simulink model "e8_IPMSM_HWJandVent_ROM"  (R2021b)
settings: Solver=VariableStepAuto  StartTime=0.0  StopTime=1000  RelTol=1e-3  AbsTol=1e-3
model workspace (MAT data in the model file):
  AdjacencyMat = [0 0 0 0 0 0 0 0 0 0 0 0 ... (15129 elements, 123x123)]
  Banding_Loss_Mat = [0 0 0 0 0 0 0 0 0 0 0 0 ... (7020 elements, 39x60x3)]
  CapMat = [1e+20 2196.70091586 387.653102799 193.8265514 1962.34710525 387.653102799 193.8265514 1962.34710525 1266.59353814 268.053957132 416.539515956 175.715078 ... (123 elements, 123x1)]
  CoolantArrayIdxs = [20 21 22 23 24 25 26 27 35 36 37 84 ... (19 elements, 19x1)]
  DCBusVoltageVec = [200 300 400]
  Friction_Loss_Mat = [0 0 0 0 0 0 0 0 0 0 0 0 ... (7020 elements, 39x60x3)]
  InletCoolIdxs = [38; 37]
  Iron_Loss_Rotor_Back_Iron_Mat = [0.0117705351991 0.0204390240307 0.0248508325185 0.0256457032681 0.0238785055856 0.020530699908 0.0166089076031 0.0132296142351 0.0115805086727 0.0121981902442 0.0144548234671 0.0172622621719 ... (7020 elements, 39x60x3)]
  Iron_Loss_Rotor_Pole_Mat = [1.45649756865 1.45220158629 1.42754923451 1.38825604934 1.33915333349 1.28386605183 1.22530180492 1.16593914393 1.10785564554 1.05188090135 0.997097257278 0.941639677474 ... (7020 elements, 39x60x3)]
  Iron_Loss_Rotor_Tooth_Mat = [0 0 0 0 0 0 0 0 0 0 0 0 ... (7020 elements, 39x60x3)]
  Iron_Loss_Stator_Back_Iron_Mat = [38.5419456951 37.7152025365 36.7151009719 35.6149517682 34.4520386289 33.2585547415 32.0665067995 30.91142079 29.8301048499 28.8255844376 27.8319778373 26.7434652419 ... (7020 elements, 39x60x3)]
  Iron_Loss_Stator_Tooth_Mat = [42.0610884508 40.9832240847 40.1258499541 39.3817529075 38.6582544091 37.9130136221 37.1370624807 36.3449214788 35.5617649366 34.7840580455 33.951564889 32.9872940506 ... (7020 elements, 39x60x3)]
  LossDistrForEachType = [0 0 0 0 0 0 0 0 0 0 0 0 ... (2952 elements, 24x123)]
  Magnet_Loss_Mat = [0.0995193918038 0.0923780277949 0.0864844160887 0.0815810725061 0.0772064600726 0.0729767275694 0.0685055432332 0.0633314716331 0.0569179480863 0.0491401889658 0.0406359949749 0.0323130751847 ... (7020 elements, 39x60x3)]
  OutletCoolIdxs = [107  107  107; 20  22  23]
  RotorCopperTempCoefResistivity = 0.00393
  Rotor_Cage_Loss_Mat = [0 0 0 0 0 0 0 0 0 0 0 0 ... (7020 elements, 39x60x3)]
  ShaftTorqueVec = [-286.936099977 -271.951133863 -256.966167748 -241.981201634 -226.99623552 -212.011269406 -197.026303292 -182.041337178 -167.056371063 -152.071404949 -137.086438835 -122.101472721 ... (39 elements, 1x39)]
  Sleeve_Loss_Mat = [0 0 0 0 0 0 0 0 0 0 0 0 ... (7020 elements, 39x60x3)]
  SpeedVec = [500 661.016949153 822.033898305 983.050847458 1144.06779661 1305.08474576 1466.10169492 1627.11864407 1788.13559322 1949.15254237 2110.16949153 2271.18644068 ... (60 elements, 1x60)]
  StateSpaceND : object (value not decoded)
  StatorCopperTempCoefResistivity = 0.00393
  Stator_Copper_Loss_AC_Mat = [0 0 0 0 0 0 0 0 0 0 0 0 ... (7020 elements, 39x60x3)]
  Stator_Copper_Loss_Mat = [3925.33912093 3478.13441392 3061.95534758 2688.26015542 2350.64396183 2044.39353286 1765.95289325 1512.57803512 1282.11615226 1072.87404999 883.521113045 712.988793321 ... (7020 elements, 39x60x3)]
  Stray_Load_Loss_Mat = [0 0 0 0 0 0 0 0 0 0 0 0 ... (7020 elements, 39x60x3)]
  Stray_Loss_Stator_Iron_Proportion = 0.95
  TnodesInit = [25 25 25 25 25 25 25 25 25 25 25 25 ... (123 elements, 123x1)]
  TrefRotor = 20
  TrefStator = 20
  Windage_Loss_Mat = [0 0 0 0 0 0 0 0 0 0 0 0 ... (7020 elements, 39x60x3)]
libraries: mcadROM_lib x4
(part 2 of 2)

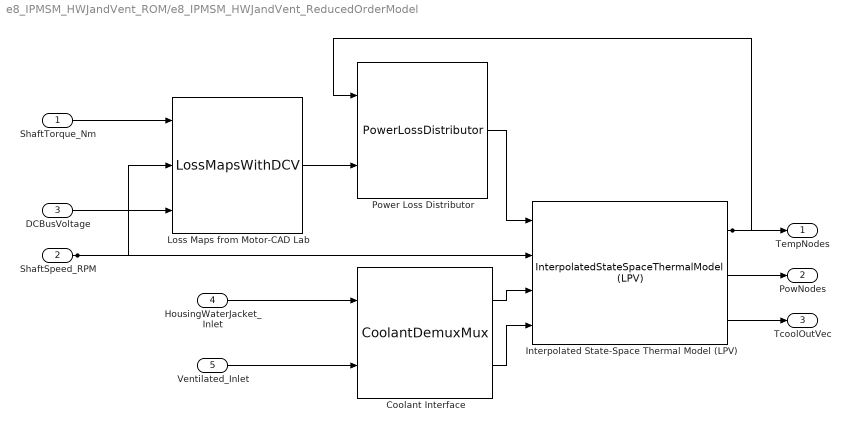
== system e8_IPMSM_HWJandVent_ROM/e8_IPMSM_HWJandVent_ReducedOrderModel ==
  ShaftTorque_Nm : Inport
  ShaftSpeed_RPM : Inport  Port=2
  DCBusVoltage : Inport  Port=3
  HousingWaterJacket_Inlet : Inport  Port=4
  Ventilated_Inlet : Inport  Port=5
  Coolant Interface : mcadROM_lib/CoolantDemuxMux  numCoolSys=2
  Interpolated State-Space Thermal Model (LPV) : mcadROM_lib/InterpolatedStateSpaceThermalModel (LPV)  StateSpaceND=StateSpaceND  CoolAdjMat=AdjacencyMat  CoolantArrayIdxs=CoolantArrayIdxs  InletCoolantIdxs=InletCoolIdxs  OutletCoolantIdxs=OutletCoolIdxs  TnodesInit=TnodesInit
  Loss Maps from Motor-CAD Lab : mcadROM_lib/LossMapsWithDCV  DCBusVoltageVec=DCBusVoltageVec  ShaftTorqueVec=ShaftTorqueVec  SpeedVec=SpeedVec  Stator_Copper_Loss_Mat=Stator_Copper_Loss_Mat  Rotor_Cage_Loss_Mat=Rotor_Cage_Loss_Mat  Iron_Loss_Stator_Back_Iron_Mat=Iron_Loss_Stator_Back_Iron_Mat  Iron_Loss_Stator_Tooth_Mat=Iron_Loss_Stator_Tooth_Mat  Stray_Loss_Stator_Iron_Proportion=Stray_Loss_Stator_Iron_Proportion  Stray_Load_Loss_Mat=Stray_Load_Loss_Mat  Magnet_Loss_Mat=Magnet_Loss_Mat  Iron_Loss_Rotor_Pole_Mat=Iron_Loss_Rotor_Pole_Mat  Iron_Loss_Rotor_Back_Iron_Mat=Iron_Loss_Rotor_Back_Iron_Mat  Iron_Loss_Rotor_Tooth_Mat=Iron_Loss_Rotor_Tooth_Mat  Friction_Loss_Mat=Friction_Loss_Mat  Windage_Loss_Mat=Windage_Loss_Mat  Stator_Copper_Loss_AC_Mat=Stator_Copper_Loss_AC_Mat  Banding_Loss_Mat=Banding_Loss_Mat  Sleeve_Loss_Mat=Sleeve_Loss_Mat
  Power Loss Distributor : mcadROM_lib/PowerLossDistributor  TrefStator=TrefStator  StatorCopperTempCoefResistivity=StatorCopperTempCoefResistivity  TrefRotor=TrefRotor  RotorCopperTempCoefResistivity=RotorCopperTempCoefResistivity  LossDistrForEachType=LossDistrForEachType  CapMat=CapMat  CoolantArrayIdxs=CoolantArrayIdxs
  TempNodes : Outport
  PowNodes : Outport  Port=2
  TcoolOutVec : Outport  Port=3
  wires:
  Interpolated State-Space Thermal Model (LPV)/1 -> Power Loss Distributor/1, TempNodes/1
  Interpolated State-Space Thermal Model (LPV)/3 -> TcoolOutVec/1
  Interpolated State-Space Thermal Model (LPV)/2 -> PowNodes/1
  Coolant Interface/2 -> Interpolated State-Space Thermal Model (LPV)/4
  Coolant Interface/1 -> Interpolated State-Space Thermal Model (LPV)/3
  Ventilated_Inlet/1 -> Coolant Interface/2
  Loss Maps from Motor-CAD Lab/1 -> Power Loss Distributor/2
  HousingWaterJacket_Inlet/1 -> Coolant Interface/1
  Power Loss Distributor/1 -> Interpolated State-Space Thermal Model (LPV)/1
  ShaftSpeed_RPM/1 -> Loss Maps from Motor-CAD Lab/2, Interpolated State-Space Thermal Model (LPV)/2
  ShaftTorque_Nm/1 -> Loss Maps from Motor-CAD Lab/1
  DCBusVoltage/1 -> Loss Maps from Motor-CAD Lab/3
